simulink model "fixed_point"  (Simulink 7.0)
settings: Solver=ode3  SolverMode=MultiTasking  StartTime=0.0  StopTime=24/3000  RelTol=1e-6
PreLoadFcn:
  | load one_stage.mat
  | load multi_stage.mat
  | load multi_stage_fixed.mat
  | generate_fir_lut
undefined symbols (not defined in the file or in its folder): hf, lut_matrix, q, quantize
libraries: simulink x10, dspmlti4 x3, simulink_extras x2, dspsigops x1
(part 2 of 2)

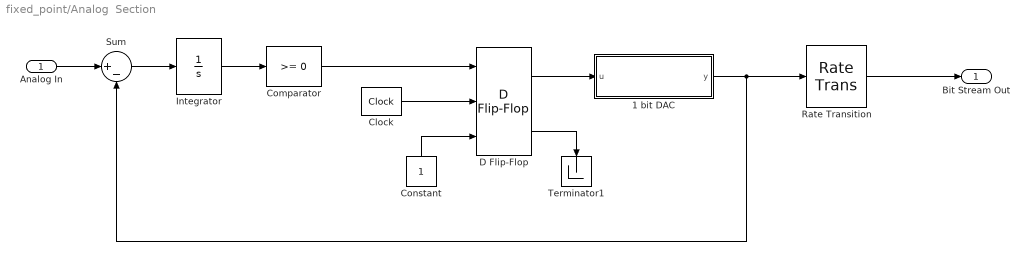
== system fixed_point/Analog  Section ==
  Analog In : Inport  OutDataType=sfix(16)  OutScaling=2^0
  1 bit DAC : Stateflow chart
  Clock : simulink_extras/Flip Flops/Clock  SystemSampleTime=-1  MaskParam1=1/(48e3*64)
  Comparator : simulink/Logic and Bit Operations/Compare To Zero  SystemSampleTime=-1  relop=>=  LogicOutDataTypeMode=boolean  ZeroCross=off
  Constant : Constant  Orientation=up  OutDataType=sfix(16)  OutScaling=2^0  SampleTime=0
  D Flip-Flop : simulink_extras/Flip Flops/D Flip-Flop  SystemSampleTime=-1
  Integrator : Integrator
  Rate Transition : RateTransition  OutPortSampleTime=1/(48e3*64)
  Sum : Sum  Inputs=|+-  OutDataType=sfix(16)  OutScaling=2^0
  Terminator1 : Terminator
      settings: Orientation=down
  Bit Stream Out : Outport  DataType=double  OutDataType=sfix(16)  OutScaling=2^0
  wires:
  Sum/1 -> Integrator/1
  Integrator/1 -> Comparator/1
  Comparator/1 -> D Flip-Flop/1
  Analog In/1 -> Sum/1
  D Flip-Flop/2 -> Terminator1/1
  D Flip-Flop/1 -> 1 bit DAC/1(u)
  Constant/1 -> D Flip-Flop/3
  1 bit DAC/1(y) -> Sum/2, Rate Transition/1
  Rate Transition/1 -> Bit Stream Out/1
  Clock/1 -> D Flip-Flop/2

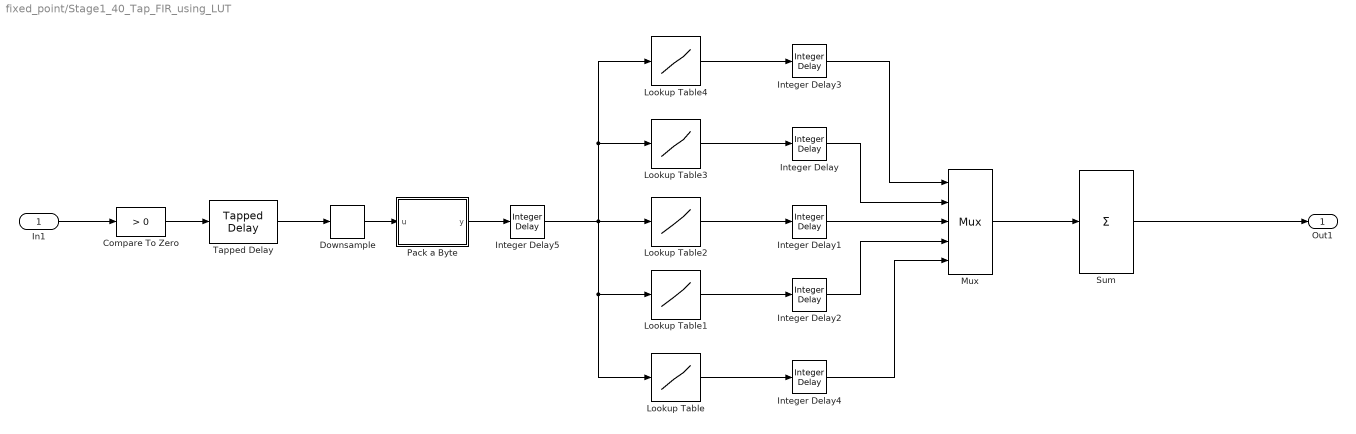
== system fixed_point/Stage1_40_Tap_FIR_using_LUT ==
  In1 : Inport  OutDataType=ufix(2)  OutScaling=2^0
  Compare To Zero : simulink/Logic and Bit Operations/Compare To Zero  SystemSampleTime=-1  relop=>  LogicOutDataTypeMode=boolean  ZeroCross=off
  Downsample : dspsigops/Downsample  N=8  phase=0  ic=0  smode=Allow multirate  fmode=Maintain input frame size
  Integer Delay : simulink/Discrete/Integer Delay  vinit=0.0  samptime=-1  NumDelays=4
  Integer Delay1 : simulink/Discrete/Integer Delay  vinit=0.0  samptime=-1  NumDelays=3
  Integer Delay2 : simulink/Discrete/Integer Delay  vinit=0.0  samptime=-1  NumDelays=2
  Integer Delay3 : simulink/Discrete/Integer Delay  vinit=0.0  samptime=-1  NumDelays=5
  Integer Delay4 : simulink/Discrete/Integer Delay  vinit=0.0  samptime=-1  NumDelays=1
  Integer Delay5 : simulink/Discrete/Integer Delay  vinit=0.0  samptime=-1  NumDelays=1
  Lookup Table : Lookup  InputValues=[0:255]  Table=quantize(q,[lut_matrix(1,:)])  OutDataTypeMode=Specify via dialog  OutDataType=fixdt(1,13,10)  RndMeth=Nearest  SaturateOnIntegerOverflow=on
  Lookup Table1 : Lookup  InputValues=[0:255]  Table=quantize(q,lut_matrix(2,:))  OutDataTypeMode=Specify via dialog  OutDataType=fixdt(1,13,10)  RndMeth=Nearest  SaturateOnIntegerOverflow=on
  Lookup Table2 : Lookup  InputValues=[0:255]  Table=quantize(q,lut_matrix(3,:))  OutDataTypeMode=Specify via dialog  OutDataType=fixdt(1,13,10)  RndMeth=Nearest  SaturateOnIntegerOverflow=on
  Lookup Table3 : Lookup  InputValues=[0:255]  Table=quantize(q,lut_matrix(4,:))  OutDataTypeMode=Specify via dialog  OutDataType=fixdt(1,13,10)  RndMeth=Nearest  SaturateOnIntegerOverflow=on
  Lookup Table4 : Lookup  InputValues=[0:255]  Table=quantize(q,lut_matrix(5,:))  OutDataTypeMode=Specify via dialog  OutDataType=fixdt(1,13,10)  RndMeth=Nearest  SaturateOnIntegerOverflow=on
  Mux : Mux  Inputs=5
  Pack a Byte : Stateflow chart
  Sum : Sum  Inputs=+  OutDataTypeMode=Specify via dialog  OutDataType=fixdt(1,13,10)  SaturateOnIntegerOverflow=on
  Tapped Delay : simulink/Discrete/Tapped Delay  vinit=0  samptime=-1  NumDelays=8  DelayOrder=Oldest  includeCurrent=off
  Out1 : Outport  OutDataType=sfix(16)  OutScaling=2^0
  wires:
  Lookup Table3/1 -> Integer Delay/1
  Lookup Table2/1 -> Integer Delay1/1
  Lookup Table1/1 -> Integer Delay2/1
  Lookup Table4/1 -> Integer Delay3/1
  In1/1 -> Compare To Zero/1
  Tapped Delay/1 -> Downsample/1
  Downsample/1 -> Pack a Byte/1(u)
  Pack a Byte/1(y) -> Integer Delay5/1
  Compare To Zero/1 -> Tapped Delay/1
  Sum/1 -> Out1/1
  Mux/1 -> Sum/1
  Integer Delay3/1 -> Mux/1
  Integer Delay/1 -> Mux/2
  Integer Delay1/1 -> Mux/3
  Integer Delay2/1 -> Mux/4
  Lookup Table/1 -> Integer Delay4/1
  Integer Delay4/1 -> Mux/5
  Integer Delay5/1 -> Lookup Table4/1, Lookup Table3/1, Lookup Table2/1, Lookup Table/1, Lookup Table1/1

== matlab function Analog Section/1 bit DAC ==
  data: u input inherited; y output inherited
function y = DAC_1_bit(u)
% This block supports an embeddable subset of the MATLAB language.
% See the help menu for details.

% This code converts boolean input to a bipolar output (double precision).
% We chose to write this in EML function block but we could have also done 
% this with simulink blocks.

y=-1+2*u;

== matlab function Stage1_40_Tap_FIR_using_LUT/Pack a Byte ==
  data: u input inherited; y output uint8
function y = fcn(u)
% This block supports an embeddable subset of the MATLAB language.
% See the help menu for details.

% This function packs eight bits into one byte.
y = uint8(0);
for k = 1:8
    y = bitset(y,k,u(k));
end
